simulink model "test_merge_funcSubsystem_output"  (R2021b)
settings: Solver=VariableStepAuto  StartTime=0.0  StopTime=10.0  RelTol=1e-3
settings Model: Creator=grodriguez  LastModifiedBy=vgaggero

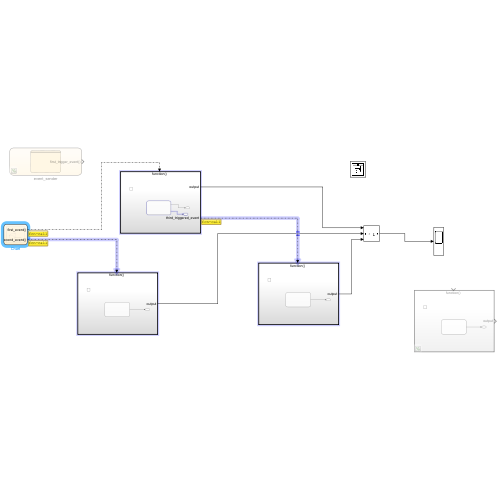
[thumbnail: Simulink's stored preview of the top-level diagram]
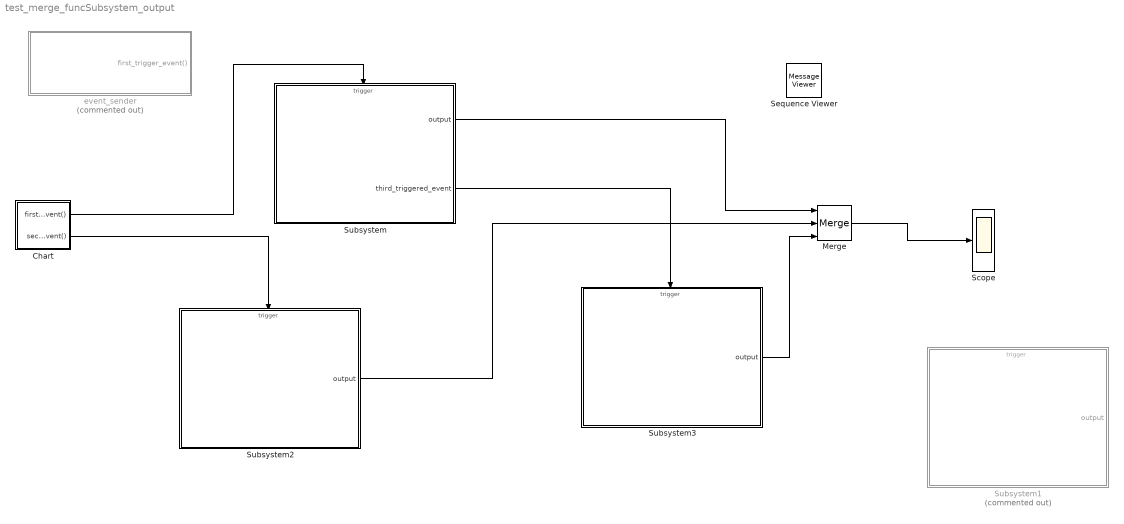
== system test_merge_funcSubsystem_output ==
  Chart : Stateflow chart  TreatAsAtomicUnit=on
  Merge : Merge  Inputs=3
  Scope : Scope
  Sequence Viewer : MessageViewer  History=1000  SavedRootId=#
  Subsystem : Subsystem
  Subsystem1 : Subsystem  Commented=on
  Subsystem2 : Subsystem
  Subsystem3 : Subsystem
  event_sender : Stateflow chart  Commented=on  TreatAsAtomicUnit=on
  wires:
  Subsystem/1(output) -> Merge/1
  Merge/1 -> Scope/1
  Chart/1(first_event()) -> Subsystem/Trigger
  Chart/2(second_event()) -> Subsystem2/Trigger
  Subsystem2/1(output) -> Merge/2
  Subsystem/2(third_triggered_event) -> Subsystem3/Trigger
  Subsystem3/1(output) -> Merge/3

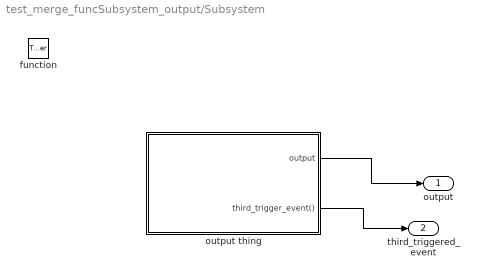
== system test_merge_funcSubsystem_output/Subsystem ==
  function : TriggerPort  TriggerType=function-call  VariantControl=(inherit)
  output thing : Stateflow chart  TreatAsAtomicUnit=on
  output : Outport
  third_triggered_event : Outport  Port=2
  wires:
  output thing/1(output) -> output/1
  output thing/2(third_trigger_event()) -> third_triggered_event/1

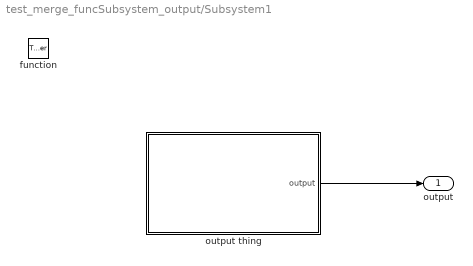
== system test_merge_funcSubsystem_output/Subsystem1 ==
  function : TriggerPort  TriggerType=function-call  VariantControl=(inherit)
  output thing : Stateflow chart  TreatAsAtomicUnit=on
  output : Outport
  wires:
  output thing/1(output) -> output/1

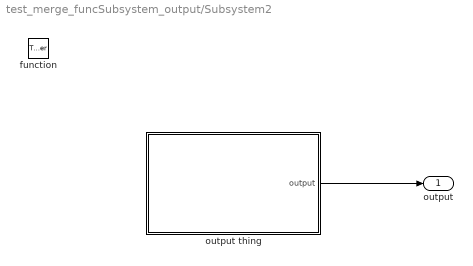
== system test_merge_funcSubsystem_output/Subsystem2 ==
  function : TriggerPort  TriggerType=function-call  VariantControl=(inherit)
  output thing : Stateflow chart  TreatAsAtomicUnit=on
  output : Outport
  wires:
  output thing/1(output) -> output/1

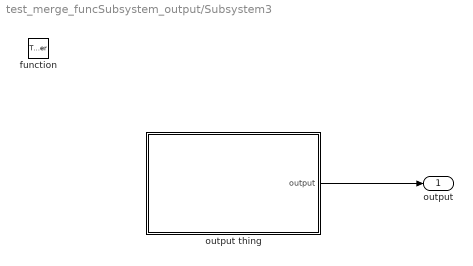
== system test_merge_funcSubsystem_output/Subsystem3 ==
  function : TriggerPort  TriggerType=function-call  VariantControl=(inherit)
  output thing : Stateflow chart  TreatAsAtomicUnit=on
  output : Outport
  wires:
  output thing/1(output) -> output/1

== stateflow chart test_merge_funcSubsystem_output/Subsystem/output thing ==
  state state_1
  state_1 -> (junction 37) [order 2] : [output<=3]
  (default) -> state_1
  (junction 37) -> state_1 : {output = output + 1;}
  state_1 -> (junction 39) [order 1] : [output>3]
  (junction 39) -> state_1 : {send(third_trigger_event);}
  data: output output =0
  events: third_trigger_event output FUNCTION_CALL_EVENT

== stateflow chart test_merge_funcSubsystem_output/Subsystem1/output thing ==
  state state_1
    entry:
    output = output + 10;
    Var1= output;
  (default) -> state_1
  data: output output =0; Var1 parameter

== stateflow chart test_merge_funcSubsystem_output/Chart ==
  state sender
    state init
      entry:
      count=count+1;
      during:
      count=count+1;
    (default) -> (junction 2)
    (junction 9) -> (junction 2)
    (junction 2) -> init
    init -> (junction 9) [order 2] : [count<=8]{send(first_event);}
    init -> (junction 9) [order 1] : [count>8]{send(second_event);}
  data: count local =0
  events: first_event output FUNCTION_CALL_EVENT; second_event output FUNCTION_CALL_EVENT

== stateflow chart test_merge_funcSubsystem_output/event_sender ==
  state first_event [parallel]
    settings: executionOrder=1
    state init
    (default) -> (junction 14)
    (junction 14) -> (junction 18)
    (junction 21) -> (junction 18)
    (junction 16) -> (junction 21)
    (junction 18) -> init : {send(first_trigger_event);}
    init -> (junction 16)
  events: first_trigger_event output FUNCTION_CALL_EVENT

== stateflow chart test_merge_funcSubsystem_output/Subsystem2/output thing ==
  state state_1
    entry:
    output = output + 10;
  (default) -> state_1
  data: output output =0

== stateflow chart test_merge_funcSubsystem_output/Subsystem3/output thing ==
  state state_1
    entry:
    output = output + 100;
  (default) -> state_1
  state_1 -> state_1
  data: output output =0
